simulink model "pre_camp"  (R2024b)
settings: Solver=VariableStepAuto  StartTime=0.0  StopTime=10.0  RelTol=1e-3
values from neighbouring files (symbols this model uses):
  g = 9.81    [pre_camp_workspace.m]
  I = eye(3,3)    [pre_camp_workspace.m]
  m = 4.34    [pre_camp_workspace.m]
settings Model: Creator=worap  LastModifiedBy=worap

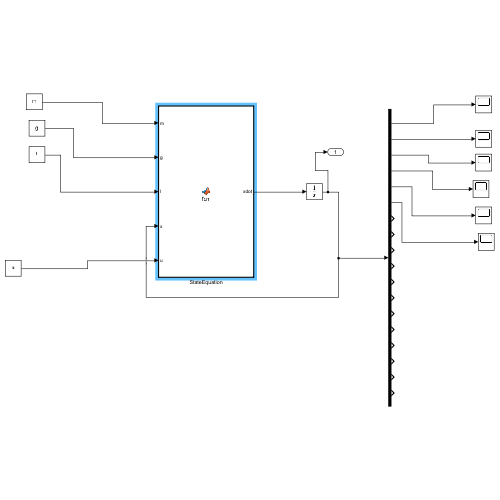
[thumbnail: Simulink's stored preview of the top-level diagram]
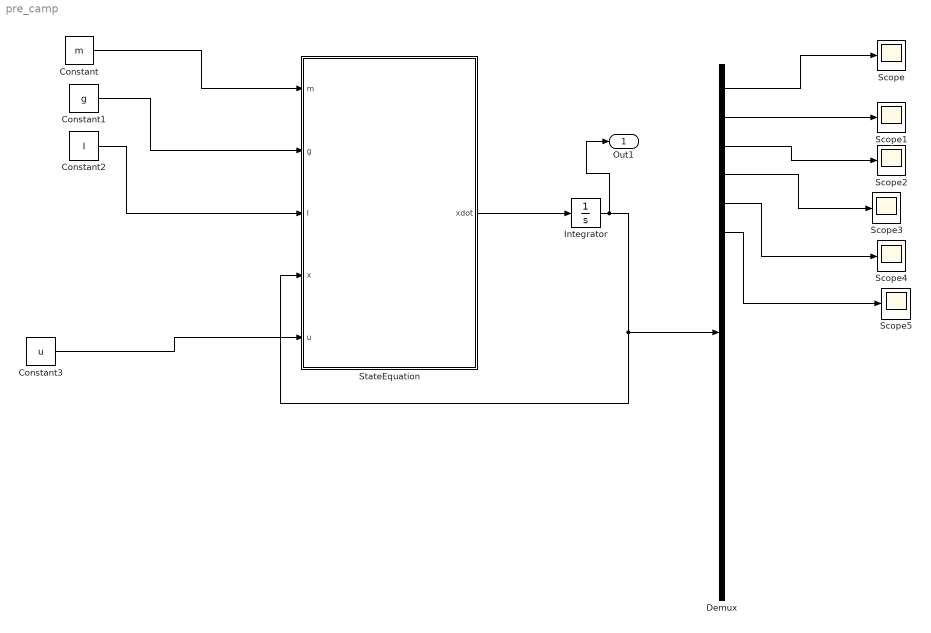
== system pre_camp ==
  Constant : Constant  Value=m
  Constant1 : Constant  Value=g
  Constant2 : Constant  Value=I
  Constant3 : Constant  Value=u
  Demux : Demux  Outputs=18
  Integrator : Integrator  InitialCondition=[0;0;0;0;0;0;1;0;0;0;1;0;0;0;1;0;0;0]
  Scope{,1..5} (6 alike) : Scope
  StateEquation : MATLAB Function  TreatAsAtomicUnit=on
  Out1 : Outport
  wires:
  Constant/1 -> StateEquation/1(m)
  Constant1/1 -> StateEquation/2(g)
  Constant2/1 -> StateEquation/3(I)
  Constant3/1 -> StateEquation/5(u)
  StateEquation/1(xdot) -> Integrator/1
  Integrator/1 -> Out1/1, StateEquation/4(x), Demux/1
  Demux/1 -> Scope/1
  Demux/2 -> Scope1/1
  Demux/3 -> Scope2/1
  Demux/4 -> Scope3/1
  Demux/5 -> Scope4/1
  Demux/6 -> Scope5/1

== matlab function pre_camp/StateEquation ==
  data: m input; g input; I input; x input; u input; xdot output
function xdot = fcn(m,g,I,x,u)

% extract the x-vextor
p = x(1:3,1);
v = x(4:6,1);
R = reshape(x(7:15,1),3,3);
omega = x(16:18,1);

%control signal
f = u(3,1);
M = u(4:6,1);

e3 = [0;0;1];


xdot = zeros(size(x));

xdot(1:3,1) = v;
xdot(4:6,1) = g*e3 - (1/m)*f*R*e3;

Rdot = R*hatmap(omega);
xdot(7:15,1) = Rdot(:);

xdot(16:18,1) = I\(M - cross(omega,I*omega));




end
